simulink model "lab4"  (R2022b)
settings: Solver=VariableStepAuto  StartTime=2  StopTime=4  RelTol=1e-3
settings Model: Creator=khrip  LastModifiedBy=mluser
settings ModelReferenceCC: EnableRefExpFcnMdlSchedulingChecks=on

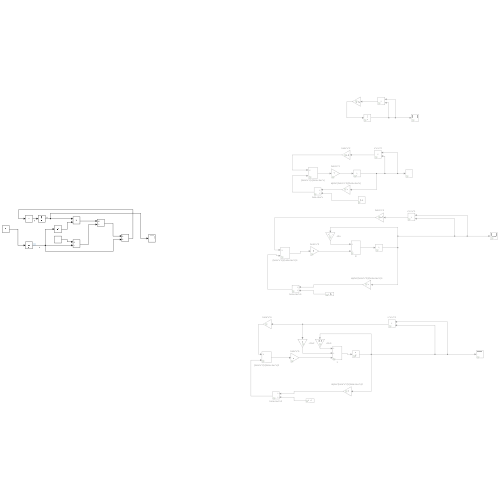
[thumbnail: Simulink's stored preview of the top-level diagram]
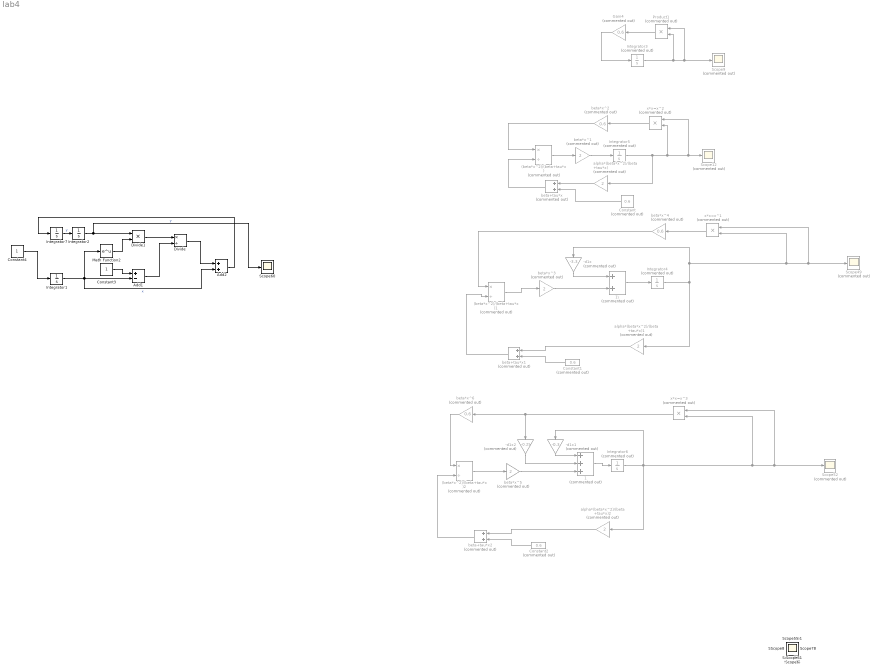
== system lab4 ==
  (beta*x^2)/(beta+tau*x) : Product  Commented=on  Inputs=*/
  (beta*x^2)/(beta+tau*x)1 : Product  Commented=on  Inputs=*/
  (beta*x^2)/(beta+tau*x)2 : Product  Commented=on  Inputs=*/
  -d1x : Gain  Commented=on  Gain=-3.3
  -d1x1 : Gain  Commented=on  Gain=-0.3
  -d1x2 : Gain  Commented=on  Gain=-0.25
  1 : Sum  Commented=on  Inputs=+++
  1\ : Sum  Commented=on
  Add1 : Sum  Inputs=+-
  Add2 : Sum
  Constant : Constant  Commented=on  Value=0.6
  Constant1 : Constant  Commented=on  Value=0.6
  Constant2 : Constant  Commented=on  Value=0.6
  Constant3 : Constant
  Constant4 : Constant
  Divide : Product  Inputs=*/
  Divide1 : Product  Inputs=**
  Gain4 : Gain  Commented=on  Gain=0.6
  Integrator1 : Integrator
  Integrator2 : Integrator
  Integrator3 : Integrator  Commented=on  InitialCondition=150*10^7
  Integrator4 : Integrator  Commented=on  InitialCondition=150*10^7
  Integrator5 : Integrator  Commented=on  InitialCondition=150*10^7
  Integrator6 : Integrator  Commented=on  InitialCondition=500
  Integrator7 : Integrator
  Math Function2 : Math
  Product1 : Product  Commented=on
  Scope{9,12,49,52} (4 alike) : Scope  Commented=on
  Scope{,1..8,10..11,13..48,50..51,53..56,58..61} (57 alike) : Scope
  alpha*(beta*x^2)/(beta+tau*x) : Gain  Commented=on  Gain=2
  alpha*(beta*x^2)/(beta+tau*x)1 : Gain  Commented=on  Gain=2
  alpha*(beta*x^2)/(beta+tau*x)2 : Gain  Commented=on  Gain=2
  beta*x^1 : Gain  Commented=on  Gain=2
  beta*x^2 : Gain  Commented=on  Gain=0.6
  beta*x^3 : Gain  Commented=on  Gain=2
  beta*x^4 : Gain  Commented=on  Gain=0.6
  beta*x^5 : Gain  Commented=on  Gain=2
  beta*x^6 : Gain  Commented=on  Gain=0.6
  beta+tau*x : Sum  Commented=on
  beta+tau*x1 : Sum  Commented=on
  beta+tau*x2 : Sum  Commented=on
  x*x=x^1 : Product  Commented=on
  x*x=x^2 : Product  Commented=on
  x*x=x^3 : Product  Commented=on
  wires:
  Product1/1 -> Gain4/1
  Integrator3/1 -> Product1/2, Product1/1, Scope9/1
  Gain4/1 -> Integrator3/1
  beta*x^2/1 -> (beta*x^2)/(beta+tau*x)/1
  Constant/1 -> beta+tau*x/2
  beta+tau*x/1 -> (beta*x^2)/(beta+tau*x)/2
  x*x=x^2/1 -> beta*x^2/1
  Integrator5/1 -> x*x=x^2/2, x*x=x^2/1, Scope12/1, alpha*(beta*x^2)/(beta+tau*x)/1
  (beta*x^2)/(beta+tau*x)/1 -> beta*x^1/1
  alpha*(beta*x^2)/(beta+tau*x)/1 -> beta+tau*x/1
  beta*x^1/1 -> Integrator5/1
  beta+tau*x1/1 -> (beta*x^2)/(beta+tau*x)1/2
  beta*x^4/1 -> (beta*x^2)/(beta+tau*x)1/1
  alpha*(beta*x^2)/(beta+tau*x)1/1 -> beta+tau*x1/1
  (beta*x^2)/(beta+tau*x)1/1 -> beta*x^3/1
  x*x=x^1/1 -> beta*x^4/1
  Constant1/1 -> beta+tau*x1/2
  Integrator4/1 -> alpha*(beta*x^2)/(beta+tau*x)1/1, x*x=x^1/2, x*x=x^1/1, Scope49/1, -d1x/1
  1\/1 -> Integrator4/1
  beta*x^3/1 -> 1\/2
  -d1x/1 -> 1\/1
  Constant2/1 -> beta+tau*x2/2
  Integrator6/1 -> x*x=x^3/2, x*x=x^3/1, Scope52/1, alpha*(beta*x^2)/(beta+tau*x)2/1, -d1x1/1
  x*x=x^3/1 -> beta*x^6/1, -d1x2/1
  (beta*x^2)/(beta+tau*x)2/1 -> beta*x^5/1
  alpha*(beta*x^2)/(beta+tau*x)2/1 -> beta+tau*x2/1
  beta*x^6/1 -> (beta*x^2)/(beta+tau*x)2/1
  -d1x1/1 -> 1/1
  beta*x^5/1 -> 1/3
  beta+tau*x2/1 -> (beta*x^2)/(beta+tau*x)2/2
  1/1 -> Integrator6/1
  -d1x2/1 -> 1/2
  Integrator1/1 -> Math Function2/1, Add1/2, Add2/2  "x"
  Integrator2/1 -> Scope60/1, Divide1/1  "y"
  Math Function2/1 -> Divide1/2
  Add1/1 -> Divide/2
  Divide1/1 -> Divide/1
  Divide/1 -> Add2/1
  Add2/1 -> Integrator7/1
  Constant3/1 -> Add1/1
  Constant4/1 -> Integrator1/1
  Integrator7/1 -> Integrator2/1  "y"
